simulink library "drivetrainLibrary"  (R2022b)
settings: Solver=VariableStepAuto  StartTime=0.0  StopTime=10.0  RelTol=1e-3
undefined symbols (not defined in the file): drivetrain
settings Model: Creator=ericb  LastModifiedBy=ericb

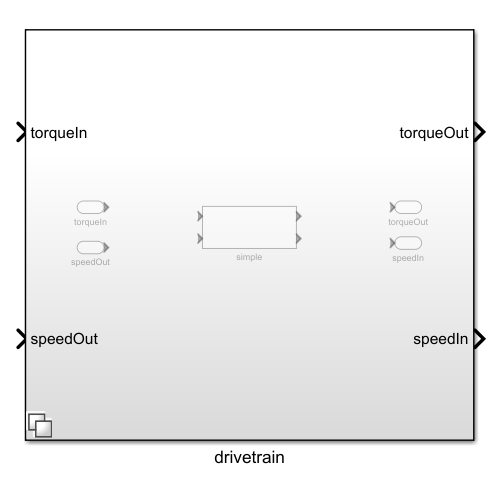
[thumbnail: Simulink's stored preview of the top-level diagram]
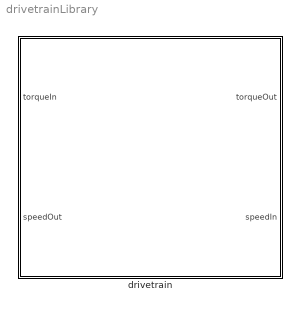
== system drivetrainLibrary ==
  drivetrain : Subsystem  Variant=on

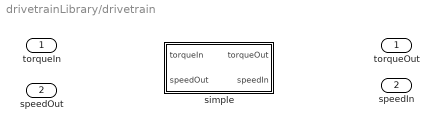
== system drivetrainLibrary/drivetrain ==
  torqueIn : Inport
  speedOut : Inport  Port=2
  simple : Subsystem  VariantControl=strcmp(drivetrain.blockChoice, 'simple')
  torqueOut : Outport
  speedIn : Outport  Port=2

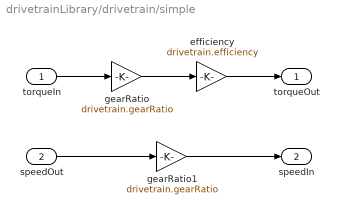
== system drivetrainLibrary/drivetrain/simple ==
  torqueIn : Inport
  speedOut : Inport  Port=2
  efficiency : Gain  Gain=drivetrain.efficiency
  gearRatio : Gain  Gain=drivetrain.gearRatio
  gearRatio1 : Gain  Gain=drivetrain.gearRatio
  torqueOut : Outport
  speedIn : Outport  Port=2
  wires:
  torqueIn/1 -> gearRatio/1
  gearRatio/1 -> efficiency/1
  efficiency/1 -> torqueOut/1
  speedOut/1 -> gearRatio1/1
  gearRatio1/1 -> speedIn/1
